simulink model "mdl_filter_kalmanIntegration2_16b"  (R2016b)
settings: Solver=ode4  StartTime=0.0  StopTime=10.0  FixedStep=Par_filterKalman.T  RelTol=1e-3  EnableMultiTasking=on
undefined symbols (not defined in the file or in its folder): Ag_phi_rad, Ag_theta_rad, AgVel_p_radPerScnd, AgVel_q_radPerScnd, DiscIntNeverNeededParam, Par_filterKalman, Par_mdlQuad, Pos_x_mtr, Pos_y_mtr, Pos_z_mtr, V_u_mtrPerScnd, V_v_mtrPerScnd, V_w_mtrPerScnd
libraries: dspstat3 x2, vrlib x1
settings Model: ExtModeTrigDuration=2  Creator=Nu  LastModifiedBy=Nu
settings OptimizationCC: MaxStackSize=64
settings DebuggingCC: ParameterTunabilityLossMsg=error
settings HardwareCC: ProdBitPerInt=16  ProdBitPerPointer=16  ProdBitPerSizeT=16  ProdBitPerPtrDiffT=16  ProdLargestAtomicFloat=None  ProdWordSize=8  ProdHWDeviceType=Atmel->AVR
settings ModelReferenceCC: ModelReferenceNumInstancesAllowed=Single
settings RTWCC: SystemTargetFile=ert.tlc  HardwareBoard=Arduino Nano 3.0  TLCOptions=-aInlineSetEventsForThisBaseRateFcn=TLC_FALSE -aSuppressMultiTaskScheduler=TLC_FALSE -aRateBasedStepFcn=1  TemplateMakefile=ert_default_tmf  Description=Embedded Coder  GenerateReport=on  Toolchain=Arduino AVR  BuildConfiguration=Faster Runs  IncludeHyperlinkInReport=on  LaunchReport=on  GenerateTraceInfo=on  GenerateTraceReport=on  GenerateTraceReportSl=on  GenerateTraceReportSf=on  GenerateTraceReportEml=on
settings CodeAppCC: ForceParamTrailComments=on  IgnoreCustomStorageClasses=off  OperatorAnnotations=on  SimulinkDataObjDesc=on  SFDataObjDesc=on  MATLABFcnDesc=on  InsertBlockDesc=on  MATLABSourceComments=on
settings ERTTargetCC: SupportContinuousTime=on  SupportVariableSizeSignals=on

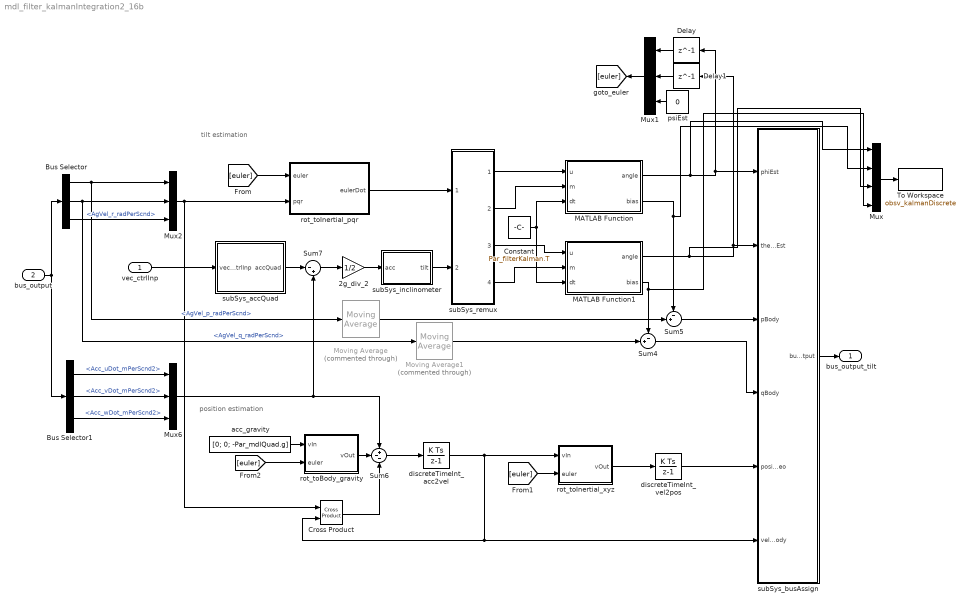
== system mdl_filter_kalmanIntegration2_16b ==
  note: position estimation
  note: tilt estimation
  vec_ctrlInp : Inport  PortDimensions=4
  bus_output : Inport  Port=2  OutDataTypeStr=Bus: mdl_output
  2g_div_2 : Gain  Gain=1/2
  Bus Selector : BusSelector  OutputSignals=AgVel_p_radPerScnd,AgVel_q_radPerScnd,AgVel_r_radPerScnd
  Bus Selector1 : BusSelector  OutputSignals=Acc_uDot_mPerScnd2,Acc_vDot_mPerScnd2,Acc_wDot_mPerScnd2
  Constant : Constant  Value=Par_filterKalman.T
  Cross Product : vrlib/Utilities/Cross Product
  Delay : Delay  DelayLength=1
  Delay1 : Delay  DelayLength=1
  MATLAB Function : MATLAB Function  TreatAsAtomicUnit=on
  MATLAB Function1 : MATLAB Function  TreatAsAtomicUnit=on
  Moving Average : dspstat3/Moving Average  Commented=through  Method=Sliding window  SpecifyWindowLength=on  WindowLength=5  ForgettingFactor=0.9  SimulateUsing=Code generation
  Moving Average1 : dspstat3/Moving Average  Commented=through  Method=Sliding window  SpecifyWindowLength=on  WindowLength=5  ForgettingFactor=0.9  SimulateUsing=Code generation
  Mux : Mux
  Mux1 : Mux  Inputs=3
  Mux2 : Mux  Inputs=3
  Mux6 : Mux  Inputs=3
  Sum4 : Sum  Inputs=-+|
  Sum5 : Sum  Inputs=-+|
  Sum6 : Sum  Inputs=+--
  Sum7 : Sum  Inputs=|-+
  To Workspace : ToWorkspace  VariableName=obsv_kalmanDiscrete  SaveFormat=Timeseries  SampleTime=-1
  acc_gravity : Constant  Value=[0; 0; -Par_mdlQuad.g]
  discreteTimeInt_acc2vel : DiscreteIntegrator  InitialConditionSetting=State (most efficient)  SampleTime=-1  ICPrevOutput=DiscIntNeverNeededParam  ICPrevScaledInput=DiscIntNeverNeededParam
  discreteTimeInt_vel2pos : DiscreteIntegrator  InitialConditionSetting=State (most efficient)  SampleTime=-1  ICPrevOutput=DiscIntNeverNeededParam  ICPrevScaledInput=DiscIntNeverNeededParam
  psiEst : Constant  Value=0
  rot_toBody_gravity : MATLAB Function  TreatAsAtomicUnit=on
  rot_toInertial_pqr : MATLAB Function  TreatAsAtomicUnit=on
  rot_toInertial_xyz : MATLAB Function  TreatAsAtomicUnit=on
  subSys_accQuad : Subsystem
  subSys_busAssign : Subsystem
  subSys_inclinometer : Subsystem
  subSys_remux : Subsystem
  "bus_output_tilt " : Outport  OutDataTypeStr=Bus: mdl_statesExt
  wires:
  bus_output/1 -> Bus Selector/1, Bus Selector1/1
  Bus Selector/3 -> Mux2/3  "<AgVel_r_radPerScnd>"
  [euler] -> rot_toInertial_pqr/1(euler)
  Bus Selector/1 -> Mux2/1, Moving Average/1  "<AgVel_p_radPerScnd>"
  Bus Selector/2 -> Mux2/2, Moving Average1/1  "<AgVel_q_radPerScnd>"
  psiEst/1 -> Mux1/3
  Sum7/1 -> 2g_div_2/1
  2g_div_2/1 -> subSys_inclinometer/1(acc)
  Mux6/1 -> Sum7/2, Sum6/1
  discreteTimeInt_acc2vel/1 -> Cross Product/2, subSys_busAssign/6(velocityBody), rot_toInertial_xyz/1(vIn)
  acc_gravity/1 -> rot_toBody_gravity/1(vIn)
  Sum6/1 -> discreteTimeInt_acc2vel/1
  rot_toBody_gravity/1(vOut) -> Sum6/2
  vec_ctrlInp/1 -> subSys_accQuad/1(vec_ctrlInp)
  subSys_accQuad/1(accQuad) -> Sum7/1
  MATLAB Function/2(bias) -> Mux/2, Sum5/1
  MATLAB Function1/2(bias) -> Mux/4, Sum4/1
  Mux1/1 -> [euler]
  [euler] -> rot_toInertial_xyz/2(euler)
  [euler] -> rot_toBody_gravity/2(euler)
  Sum5/1 -> subSys_busAssign/3(pBody)
  Sum4/1 -> subSys_busAssign/4(qBody)
  discreteTimeInt_vel2pos/1 -> subSys_busAssign/5(positionGeo)
  subSys_busAssign/1(bus_output) -> "bus_output_tilt "/1
  Bus Selector1/1 -> Mux6/1  "<Acc_uDot_mPerScnd2>"
  Bus Selector1/2 -> Mux6/2  "<Acc_vDot_mPerScnd2>"
  Bus Selector1/3 -> Mux6/3  "<Acc_wDot_mPerScnd2>"
  rot_toInertial_pqr/1(eulerDot) -> subSys_remux/1(eulerDot)
  subSys_inclinometer/1(tilt) -> subSys_remux/2(euler)
  subSys_remux/1(phiDot) -> MATLAB Function/1(u)
  subSys_remux/2(phiEst) -> MATLAB Function/2(m)
  subSys_remux/4(thetaEst) -> MATLAB Function1/2(m)
  Moving Average/1 -> Sum5/2
  Moving Average1/1 -> Sum4/2
  rot_toInertial_xyz/1(vOut) -> discreteTimeInt_vel2pos/1
  Mux2/1 -> rot_toInertial_pqr/2(pqr), Cross Product/1
  Cross Product/1 -> Sum6/3
  subSys_remux/3(thetaDot) -> MATLAB Function1/1(u)
  Constant/1 -> MATLAB Function1/3(dt), MATLAB Function/3(dt)
  MATLAB Function/1(angle) -> Mux/1, Delay/1, subSys_busAssign/1(phiEst)
  MATLAB Function1/1(angle) -> Mux/3, Delay1/1, subSys_busAssign/2(thetaEst)
  Delay/1 -> Mux1/1
  Delay1/1 -> Mux1/2
  Mux/1 -> To Workspace/1

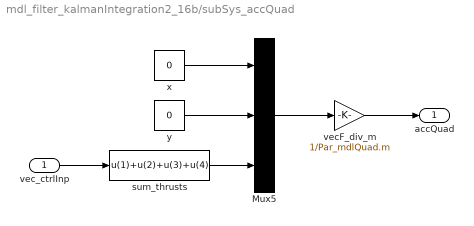
== system mdl_filter_kalmanIntegration2_16b/subSys_accQuad ==
  vec_ctrlInp : Inport
  Mux5 : Mux  Inputs=3
  sum_thrusts : Fcn  Expr=u(1)+u(2)+u(3)+u(4)
  vecF_div_m : Gain  Gain=1/Par_mdlQuad.m
  x : Constant  Value=0
  y : Constant  Value=0
  accQuad : Outport
  wires:
  sum_thrusts/1 -> Mux5/3
  x/1 -> Mux5/1
  y/1 -> Mux5/2
  vecF_div_m/1 -> accQuad/1
  Mux5/1 -> vecF_div_m/1
  vec_ctrlInp/1 -> sum_thrusts/1

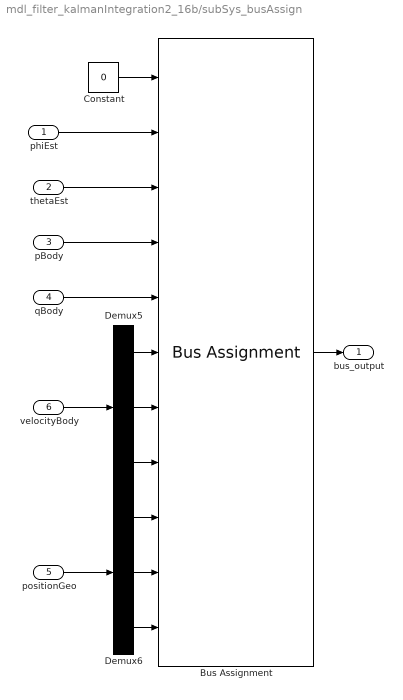
== system mdl_filter_kalmanIntegration2_16b/subSys_busAssign ==
  phiEst : Inport
  thetaEst : Inport  Port=2
  pBody : Inport  Port=3
  qBody : Inport  Port=4
  positionGeo : Inport  Port=5
  velocityBody : Inport  Port=6
  Bus Assignment : BusAssignment  AssignedSignals=Ag_phi_rad,Ag_theta_rad,AgVel_p_radPerScnd,AgVel_q_radPerScnd,V_u_mtrPerScnd,V_v_mtrPerScnd,V_w_mtrPerScnd,Pos_x_mtr,Pos_y_mtr,Pos_z_mtr
  Constant : Constant  Value=0  OutDataTypeStr=Bus: mdl_statesExt
  Demux5 : Demux  Outputs=3
  Demux6 : Demux  Outputs=3
  bus_output : Outport
  wires:
  velocityBody/1 -> Demux5/1
  phiEst/1 -> Bus Assignment/2
  thetaEst/1 -> Bus Assignment/3
  Constant/1 -> Bus Assignment/1
  qBody/1 -> Bus Assignment/5
  Bus Assignment/1 -> bus_output/1
  Demux5/1 -> Bus Assignment/6
  positionGeo/1 -> Demux6/1
  Demux6/1 -> Bus Assignment/9
  Demux5/3 -> Bus Assignment/8
  Demux6/2 -> Bus Assignment/10
  Demux5/2 -> Bus Assignment/7
  Demux6/3 -> Bus Assignment/11
  pBody/1 -> Bus Assignment/4

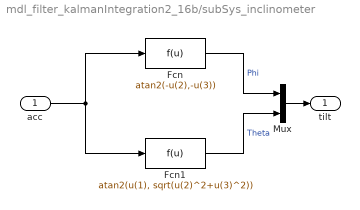
== system mdl_filter_kalmanIntegration2_16b/subSys_inclinometer ==
  acc : Inport
  Fcn : Fcn  Expr=atan2(-u(2),-u(3))
  Fcn1 : Fcn  Expr=atan2(u(1), sqrt(u(2)^2+u(3)^2))
  Mux : Mux  Inputs=2
  tilt : Outport
  wires:
  acc/1 -> Fcn/1, Fcn1/1
  Fcn/1 -> Mux/1  "Phi"
  Fcn1/1 -> Mux/2  "Theta"
  Mux/1 -> tilt/1

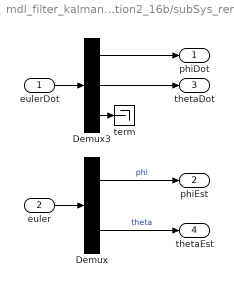
== system mdl_filter_kalmanIntegration2_16b/subSys_remux ==
  eulerDot : Inport
  euler : Inport  Port=2
  Demux : Demux  Outputs=2
  Demux3 : Demux  Outputs=3
  term : Terminator
  phiDot : Outport
  phiEst : Outport  Port=2
  thetaDot : Outport  Port=3
  thetaEst : Outport  Port=4
  wires:
  eulerDot/1 -> Demux3/1
  Demux3/3 -> term/1
  euler/1 -> Demux/1
  Demux3/1 -> phiDot/1
  Demux/2 -> thetaEst/1  "theta"
  Demux/1 -> phiEst/1  "phi"
  Demux3/2 -> thetaDot/1

== matlab function mdl_filter_kalmanIntegration2_16b/rot_toInertial_xyz ==
  data: vIn input; euler input; vOut output
function vOut = fcn(vIn, euler)

vOut = rot_euler(vIn, euler, 'to-inertial-frame');

== matlab function mdl_filter_kalmanIntegration2_16b/rot_toBody_gravity ==
  data: vIn input; euler input; vOut output
function vOut = fcn(vIn, euler)

vOut = rot_euler(vIn, euler, 'to-body-frame');

== matlab function mdl_filter_kalmanIntegration2_16b/MATLAB Function ==
  data: u input; angle output; m input; dt input; bias output
function [angle, bias]= kalman(u,m,dt)
%%%%%%%%%%%%%%%%%%%%%%%%%%%%%%%%%%%%%%%%%%%%%%%%%%%%%%%%%%%%%%%%%%%%%%%%%%%
% Kalman filter implementation for gyroscope and accelerometer sensor
% fusion.
% Based on the system model:
%
% x_k = F*x_k-1 + B*u_k + w_k
%
% where:
%
% x_k =[angle]    F = [1 -dt]                 B = [dt]
%      [bias ]        [0  1 ]                     [0 ]
% Sytem states    State transition matrix     Control input matrix
% 
% w_k - Process noise            Q_k = [Q_angle    0  ]
%                                      [   0    Q_bias]
%                                Process noise covariance matrix
% and the measurement model:
%
% z_k = H*x_k + v_k
%
% where:
%
% H = [1 0]             v_k - Measurement noise      R = var(v_k)
% Observation matrix                                 Measurement noise 
%                                                    covariance matrix 
persistent P x_hat F B H Q R
if isempty(P)
    % Initialization at first run
    Q_angle = 0.001; % Variance of the estimated gyro angle
    Q_bias = 0.003;  % Variance of the bias estimation
    angle_0 = 0;     % Initial angle guess
    bias_0 = 0;      % Reset bias as we assume we know the initial
                     % state of the system and do a calibration routine
    P = zeros(2,2);  % Error covariance matrix is set to zero, since we
                     % assume we know the initial state and bias
    x_hat = [angle_0 bias_0]';  % Initial state vector
    F = [1 -dt; 0 1];           % State transition matrix
    B = [dt 0]';                % Input matrix
    Q = diag([Q_angle Q_bias]); % Process noise covariance matrix
    H = [1 0];                  % Observation model
    R = 0.8;                    % Measurement variance
end
%%%%%%%%%%%%%%%%%%%%%%%%%%%%%%%%%%%%%%%%%%%%%%%%%%%%%%%%%%%%%%%%%%%%%%%%%%%
% Kalman filter algorithm
% Prediction:
%
% Step 1: Update x_hat - predict next state
x_hat = F*x_hat + B*u;
% Step 2: Update error covariance matrix
P = F*P*F' + Q;
% Correction:
%
% Step 3: Calculate the kalman gain
K = P*H'/(H*P*H' + R);
% Step 4: Calculate measurement residual
y_r = m - H*x_hat;
% Step 5: Update the state and error covariance
x_hat = x_hat + K*y_r;
P = (eye(2,2)-K*H)*P;
% Output the result
angle = x_hat(1);
bias = x_hat(2);

== matlab function mdl_filter_kalmanIntegration2_16b/MATLAB Function1 ==
  data: u input; angle output; m input; dt input; bias output
function [angle, bias]= kalman(u,m,dt)
%%%%%%%%%%%%%%%%%%%%%%%%%%%%%%%%%%%%%%%%%%%%%%%%%%%%%%%%%%%%%%%%%%%%%%%%%%%
% Kalman filter implementation for gyroscope and accelerometer sensor
% fusion.
% Based on the system model:
%
% x_k = F*x_k-1 + B*u_k + w_k
%
% where:
%
% x_k =[angle]    F = [1 -dt]                 B = [dt]
%      [bias ]        [0  1 ]                     [0 ]
% Sytem states    State transition matrix     Control input matrix
% 
% w_k - Process noise            Q_k = [Q_angle    0  ]
%                                      [   0    Q_bias]
%                                Process noise covariance matrix
% and the measurement model:
%
% z_k = H*x_k + v_k
%
% where:
%
% H = [1 0]             v_k - Measurement noise      R = var(v_k)
% Observation matrix                                 Measurement noise 
%                                                    covariance matrix 
persistent P x_hat F B H Q R
if isempty(P)
    % Initialization at first run
    Q_angle = 0.001; % Variance of the estimated gyro angle
    Q_bias = 0.003;  % Variance of the bias estimation
    angle_0 = 0;     % Initial angle guess
    bias_0 = 0;      % Reset bias as we assume we know the initial
                     % state of the system and do a calibration routine
    P = zeros(2,2);  % Error covariance matrix is set to zero, since we
                     % assume we know the initial state and bias
    x_hat = [angle_0 bias_0]';  % Initial state vector
    F = [1 -dt; 0 1];           % State transition matrix
    B = [dt 0]';                % Input matrix
    Q = diag([Q_angle Q_bias]); % Process noise covariance matrix
    H = [1 0];                  % Observation model
    R = 0.8;                    % Measurement variance
end
%%%%%%%%%%%%%%%%%%%%%%%%%%%%%%%%%%%%%%%%%%%%%%%%%%%%%%%%%%%%%%%%%%%%%%%%%%%
% Kalman filter algorithm
% Prediction:
%
% Step 1: Update x_hat - predict next state
x_hat = F*x_hat + B*u;
% Step 2: Update error covariance matrix
P = F*P*F' + Q;
% Correction:
%
% Step 3: Calculate the kalman gain
K = P*H'/(H*P*H' + R);
% Step 4: Calculate measurement residual
y_r = m - H*x_hat;
% Step 5: Update the state and error covariance
x_hat = x_hat + K*y_r;
P = (eye(2,2)-K*H)*P;
% Output the result
angle = x_hat(1);
bias = x_hat(2);

== matlab function mdl_filter_kalmanIntegration2_16b/rot_toInertial_pqr ==
  data: euler input; eulerDot output; pqr input
function eulerDot = fcn(euler, pqr)

eulerDot = rot_karman(pqr, euler, 'to-inertial-frame');
